simulink subsystem "ACC_Controller"  (R2024b)
settings: Solver=VariableStepAuto  StartTime=0.0  StopTime=10.0  RelTol=1e-3
libraries: mpcadaslib x1
settings Model: Creator=Tong  LastModifiedBy=Tong

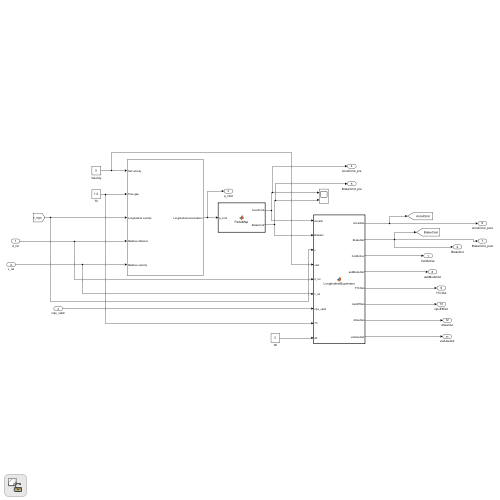
[thumbnail: Simulink's stored preview of the top-level diagram]
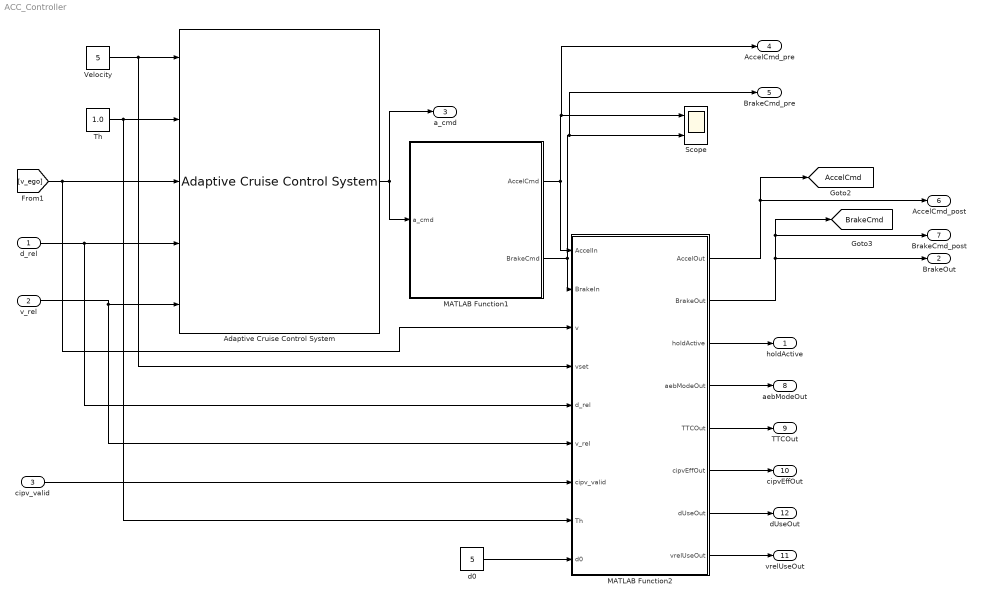
== system ACC_Controller ==
  d_rel : Inport
  v_rel : Inport  Port=2
  cipv_valid : Inport  Port=3
  Adaptive Cruise Control System : mpcadaslib/Adaptive Cruise Control System  EgoModel=tf(1,[0.5,1,0])  InitialEgoVelocity=5  DefaultSpacing=5  MaxVelocity=50  MinAcceleration=-2  amin_ext=off  MaxAcceleration=2  amax_ext=off  Ts=0.05  PredictionHorizon=30  ControllerBehavior=0.600  suboptimal=off  maxiter=10  datatypeopt=double  optmode=off  trackmode=off
      settings: LibrarySourceBlock=mpclib/Automated Driving/Adaptive Cruise Control System
  MATLAB Function1 : MATLAB Function  TreatAsAtomicUnit=on
  MATLAB Function2 : MATLAB Function  TreatAsAtomicUnit=on
  Scope : Scope  NumInputPorts=2
  Th : Constant  Value=1.0
  Velocity : Constant  Value=5
  d0 : Constant  Value=5
  holdActive : Outport
  BrakeOut : Outport  Port=2
  a_cmd : Outport  Port=3
  AccelCmd_pre : Outport  Port=4
  BrakeCmd_pre : Outport  Port=5
  AccelCmd_post : Outport  Port=6
  BrakeCmd_post : Outport  Port=7
  aebModeOut : Outport  Port=8
  TTCOut : Outport  Port=9
  cipvEffOut : Outport  Port=10
  vrelUseOut : Outport  Port=11
  dUseOut : Outport  Port=12
  tag scope: AccelCmd=global, BrakeCmd=global
  wires:
  d_rel/1 -> Adaptive Cruise Control System/4, MATLAB Function2/5(d_rel)
  v_rel/1 -> Adaptive Cruise Control System/5, MATLAB Function2/6(v_rel)
  [v_ego] -> Adaptive Cruise Control System/3, MATLAB Function2/3(v)
  Adaptive Cruise Control System/1 -> MATLAB Function1/1(a_cmd), a_cmd/1
  Th/1 -> Adaptive Cruise Control System/2, MATLAB Function2/8(Th)
  MATLAB Function1/1(AccelCmd) -> MATLAB Function2/1(AccelIn), Scope/1, AccelCmd_pre/1
  MATLAB Function1/2(BrakeCmd) -> MATLAB Function2/2(BrakeIn), Scope/2, BrakeCmd_pre/1
  MATLAB Function2/1(AccelOut) -> AccelCmd_post/1, [AccelCmd]
  MATLAB Function2/2(BrakeOut) -> BrakeOut/1, BrakeCmd_post/1, [BrakeCmd]
  Velocity/1 -> Adaptive Cruise Control System/1, MATLAB Function2/4(vset)
  d0/1 -> MATLAB Function2/9(d0)
  cipv_valid/1 -> MATLAB Function2/7(cipv_valid)
  MATLAB Function2/3(holdActive) -> holdActive/1
  MATLAB Function2/4(aebModeOut) -> aebModeOut/1
  MATLAB Function2/5(TTCOut) -> TTCOut/1
  MATLAB Function2/6(cipvEffOut) -> cipvEffOut/1
  MATLAB Function2/7(dUseOut) -> dUseOut/1
  MATLAB Function2/8(vrelUseOut) -> vrelUseOut/1

== matlab function ACC_Controller/MATLAB Function1 ==
  settings: updateMethod=DISCRETE
  data: a_cmd input; AccelCmd output; BrakeCmd output
function [AccelCmd, BrakeCmd] = PedalMap(a_cmd)
%#codegen
% a_cmd: desired longitudinal acceleration (m/s^2)
% outputs: AccelCmd/BrakeCmd in [0,1]

% === 需要按你的模型改的参数 ===
Ts = 0.05;        % 采样时间：与你Supervisor一致就行
aAccelMax = 2.0;  % 认为“满油门”对应的加速度 (m/s^2)
aBrakeMax = 4.0;  % 认为“满刹车”对应的减速度幅值 (m/s^2)
aDead = 0.08;     % 加速度死区 (m/s^2)，抑制0附近抖动：0.05~0.15可调

% 软启动非线性：>1 更温和（小命令更小踏板）
gammaAcc = 1.4;
gammaBrk = 1.2;

% 踏板变化率限制（每秒最大变化量）
pedalRate = 3.5;  % 1/s，越大越“灵”，越小越平顺（1.5~4可调）
dPed = pedalRate * Ts;

persistent accPrev brkPrev
if isempty(accPrev)
    accPrev = 0;
    brkPrev = 0;
end

% --- 1) 死区 + 归一化 ---
acc = 0;
brk = 0;

if a_cmd > aDead
    x = (a_cmd - aDead) / max(aAccelMax - aDead, 1e-3);
    x = min(max(x, 0), 1);
    acc = x^gammaAcc;
elseif a_cmd < -aDead
    x = (-a_cmd - aDead) / max(aBrakeMax - aDead, 1e-3);
    x = min(max(x, 0), 1);
    brk = x^gammaBrk;
end

% --- 2) 变化率限制（避免踏板突跳） ---
acc = min(max(acc, accPrev - dPed), accPrev + dPed);
brk = min(max(brk, brkPrev - dPed), brkPrev + dPed);

% --- 3) 互斥（稳妥，避免同时给油/给刹） ---
if brk > 0
    acc = 0;
elseif acc > 0
    brk = 0;
end

% --- 4) 限幅并更新 ---
AccelCmd = min(max(acc, 0), 1);
BrakeCmd = min(max(brk, 0), 1);

accPrev = AccelCmd;
brkPrev = BrakeCmd;
end

== matlab function ACC_Controller/MATLAB Function2 ==
  data: AccelIn input; AccelOut output; BrakeIn input; v input; vset input; d_rel input; v_rel input; cipv_valid input; Th input; d0 input; BrakeOut output; holdActive output; aebModeOut output; TTCOut output; cipvEffOut output; dUseOut output; vrelUseOut output
function [AccelOut, BrakeOut, holdActive, aebModeOut, TTCOut, cipvEffOut, dUseOut, vrelUseOut] = ...
    LongitudinalSupervisor(AccelIn, BrakeIn, v, vset, d_rel, v_rel, cipv_valid, Th, d0)
%#codegen
% LongitudinalSupervisor - Paper Mode
%
% 输入:
%   AccelIn, BrakeIn - 上游加速/制动命令，0~1
%   v                - ego 纵向速度，m/s
%   vset             - 设定速度，m/s
%   d_rel            - 真值相对距离，m
%   v_rel            - 真值相对速度，lead - ego，接近时为负
%   cipv_valid       - 上游目标有效标志
%   Th               - 时距
%   d0               - 最小间距
%
% 输出:
%   AccelOut, BrakeOut - 最终踏板命令
%   holdActive         - 停车保持状态
%   aebModeOut         - 0 none, 1 FCW, 2 PB1, 3 FB
%   TTCOut             - TTC
%   cipvEffOut         - Supervisor 实际采用的目标有效性
%   dUseOut            - Supervisor 实际使用距离
%   vrelUseOut         - Supervisor 实际使用相对速度

%% ================= 参数区 =================
TTC_MAX = 1e6;
NO_TARGET_DIST = 199.5;

% 论文模式：直接用真值距离/速度判断目标
USE_TRUTH_CONTROL = true;

% 目标丢失短时保持
Ts = 0.05;
t_drop_hold = 0.5;
N_drop = int32(round(t_drop_hold / Ts));

% ACC 安全距离
margin = 2.0;

% TTC 阈值
FCWtime = 1.8;
PB1time = 1.1;
FBtime  = 0.7;
TimeFactor = 1.3;
N_on = int32(2);

% 制动强度
PB1_brake = 0.25;
FB_brake  = 0.80;
EMG_brake = 1.00;

% 极近距离保护
d_emg = 1.5;

% 低速停车保持
v_hold = 0.25;
d_hold = d0 + 0.8;
d_relax = d0 + 2.0;
vrel_release = 0.15;

% 低速非紧急制动限幅，避免低速抖动太难看
v_low_brk_cap = 1.0;
brake_lowspd_cap = 0.45;

% 相对速度死区
if abs(v_rel) < 0.15
    v_rel = 0.0;
end

%% ================= 持久变量 =================
persistent haveLast lostCnt dLast vrelLast
persistent hold
persistent cntClosing aebMode

if isempty(haveLast)
    haveLast = false;
    lostCnt = int32(0);
    dLast = 200.0;
    vrelLast = 0.0;
end

if isempty(hold)
    hold = false;
end

if isempty(cntClosing)
    cntClosing = int32(0);
end

if isempty(aebMode)
    aebMode = int32(0);
end

%% ================= 1. 目标有效性与使用值 =================
if USE_TRUTH_CONTROL
    rawValid = (d_rel > 0.0) && (d_rel < NO_TARGET_DIST);

    if rawValid
        cipv_eff = true;
        d_use = d_rel;
        vrel_use = v_rel;

        haveLast = true;
        lostCnt = int32(0);
        dLast = d_use;
        vrelLast = vrel_use;
    else
        % 真值短时丢失时，保持上一帧，避免曲线突然跳 200
        if haveLast && (lostCnt < N_drop)
            lostCnt = lostCnt + 1;
            cipv_eff = true;
            d_use = dLast;
            vrel_use = vrelLast;
        else
            cipv_eff = false;
            d_use = 200.0;
            vrel_use = 0.0;

            haveLast = false;
            lostCnt = int32(0);
            dLast = 200.0;
            vrelLast = 0.0;
        end
    end
else
    % 原始模式：依赖 cipv_valid
    if cipv_valid > 0.5
        cipv_eff = true;
        d_use = d_rel;
        vrel_use = v_rel;

        haveLast = true;
        lostCnt = int32(0);
        dLast = d_use;
        vrelLast = vrel_use;
    else
        if haveLast && (lostCnt < N_drop)
            lostCnt = lostCnt + 1;
            cipv_eff = true;
            d_use = dLast;
            vrel_use = vrelLast;
        else
            cipv_eff = false;
            d_use = 200.0;
            vrel_use = 0.0;

            haveLast = false;
            lostCnt = int32(0);
        end
    end
end

%% ================= 2. 期望距离与 TTC =================
d_ref = d0 + Th * v;

closing = cipv_eff && (d_use > 0.0) && (vrel_use < -0.2) && (v > 0.3);

if closing
    TTC = d_use / (-vrel_use);
    if TTC > TTC_MAX
        TTC = TTC_MAX;
    end
else
    TTC = TTC_MAX;
end

TTCOut = TTC;

%% ================= 3. Stop & Hold =================
if (~hold) && cipv_eff && (v < v_hold) && (d_use < d_hold)
    hold = true;
end

if hold
    if (~cipv_eff) || ...
       ((vrel_use > vrel_release) && (d_use > d_relax)) || ...
       (d_use > d_ref + 1.0)
        hold = false;
    end
end

holdActive = hold;

%% ================= 4. AEB 状态机 =================
if closing && (TTC < FCWtime)
    cntClosing = min(cntClosing + 1, int32(100));
else
    cntClosing = int32(0);
end

closingStable = cntClosing >= N_on;

switch aebMode
    case 0
        if closingStable && (TTC < FCWtime)
            aebMode = int32(1);
        end

    case 1
        if (~closing) || (TTC > TimeFactor * FCWtime)
            aebMode = int32(0);
        elseif TTC < PB1time
            aebMode = int32(2);
        end

    case 2
        if (~closing) || (TTC > TimeFactor * PB1time)
            aebMode = int32(0);
        elseif TTC < FBtime
            aebMode = int32(3);
        end

    otherwise
        if (~closing) || (TTC > TimeFactor * FBtime)
            aebMode = int32(0);
        end
end

%% ================= 5. 输出优先级 =================
AccelOut = AccelIn;
BrakeOut = BrakeIn;

isEmergency = cipv_eff && (d_use < d_emg);

if isEmergency
    AccelOut = 0.0;
    BrakeOut = EMG_brake;

elseif hold
    AccelOut = 0.0;
    BrakeOut = EMG_brake;

else
    % AEB 分级
    if aebMode == 1
        AccelOut = 0.0;

    elseif aebMode == 2
        AccelOut = 0.0;
        if BrakeOut < PB1_brake
            BrakeOut = PB1_brake;
        end

    elseif aebMode == 3
        AccelOut = 0.0;
        if BrakeOut < FB_brake
            BrakeOut = FB_brake;
        end
    end

    % 安全距离内且正在接近：禁止继续加速
    if cipv_eff && (d_use < d_ref + margin) && (vrel_use < -0.1)
        AccelOut = 0.0;

        % 给一点温和制动，让图上能体现监督层介入
        if BrakeOut < 0.10
            BrakeOut = 0.10;
        end
    end

    % 没有目标时，不主动覆盖上游制动；只防止小残余刹车长期存在
    if (~cipv_eff) && (BrakeOut < 0.03)
        BrakeOut = 0.0;
    end

    % 低速下非 FB 不要太猛
    if (v < v_low_brk_cap) && (aebMode < 3) && (~isEmergency)
        if BrakeOut > brake_lowspd_cap
            BrakeOut = brake_lowspd_cap;
        end
    end
end

%% ================= 6. 加速制动互斥 =================
if (BrakeOut > 0.001) && (AccelOut > 0.001)
    if BrakeOut >= AccelOut
        AccelOut = 0.0;
    else
        BrakeOut = 0.0;
    end
end

%% ================= 7. 限幅 =================
if AccelOut < 0.0
    AccelOut = 0.0;
elseif AccelOut > 1.0
    AccelOut = 1.0;
end

if BrakeOut < 0.0
    BrakeOut = 0.0;
elseif BrakeOut > 1.0
    BrakeOut = 1.0;
end

%% ================= 8. 日志输出 =================
aebModeOut = double(aebMode);
cipvEffOut = double(cipv_eff);
dUseOut = d_use;
vrelUseOut = vrel_use;

end


% function [AccelOut, BrakeOut, holdActive, aebModeOut, TTCOut, cipvEffOut, dUseOut, vrelUseOut] = ...
%     LongitudinalSupervisor(AccelIn, BrakeIn, v, vset, d_rel, v_rel, cipv_valid, Th, d0)
% %#codegen
% % LongitudinalSupervisor (0~1 pedal commands)
% % v_rel 定义：lead - ego（接近时 v_rel<0）
% 
% %% ========== 采样时间 ==========
% Ts = 0.05;
% 
% %% ========== 参数区（可调） ==========
% epsV   = 0.2;
% margin = 2.0;
% K_over = 0.35;
% 
% v_hold       = 0.3;
% d_hold       = d0 + 0.8;
% d_relax      = d0 + 2.0;
% vrel_release = 0.15;
% relax_by_ref = 1.0;
% 
% d_emg = 1.5;
% 
% t_drop_hold = 0.5;
% N_drop = int32(round(t_drop_hold/Ts));
% 
% v_low_brk_cap    = 1.0;
% brake_lowspd_cap = 0.35;
% 
% if abs(v_rel) < 0.2
%     v_rel = 0;
% end
% 
% FCWtime    = 1.8;
% PB1time    = 1.1;
% FBtime     = 0.7;
% TimeFactor = 1.3;
% N_on       = int32(3);
% PB1_brake_min = 0.15;
% 
% %% ========== 期望距离 ==========
% d_ref = d0 + Th*v;
% 
% %% ========== 目标丢失保持 ==========
% persistent lostCnt haveLast dLast vrelLast
% if isempty(haveLast)
%     lostCnt  = int32(0);
%     haveLast = false;
%     dLast    = 200;
%     vrelLast = 0;
% end
% 
% if cipv_valid > 0.5
%     haveLast = true;
%     lostCnt  = int32(0);
%     dLast    = d_rel;
%     vrelLast = v_rel;
%     cipv_eff = true;
%     d_use    = d_rel;
%     vrel_use = v_rel;
% else
%     if haveLast && (lostCnt < N_drop)
%         lostCnt  = lostCnt + 1;
%         cipv_eff = true;
%         d_use    = dLast;
%         vrel_use = vrelLast;
%     else
%         cipv_eff = false;
%         d_use    = d_rel;
%         vrel_use = v_rel;
%         haveLast = false;
%     end
% end
% 
% %% ========== Stop&Hold 状态机 ==========
% persistent hold
% if isempty(hold), hold = false; end
% 
% if (~hold) && cipv_eff && (v < v_hold) && (d_use < d_hold)
%     hold = true;
% end
% 
% if hold
%     if (~cipv_eff) || ...
%        ((vrel_use > vrel_release) && (d_use > d_relax)) || ...
%        (d_use > d_ref + relax_by_ref)
%         hold = false;
%     end
% end
% 
% holdActive = hold;
% 
% %% ========== TTC分级状态机 ==========
% closing = cipv_eff && (vrel_use < -0.2) && (d_use > 0) && (v > 0.5);
% % if closing
% %     TTC = d_use / (-vrel_use);
% % else
% %     TTC = inf;
% % end
% 
% TTC_MAX = 1e6;
% if closing && (-vrel_use > 1e-3)
%     TTC = d_use / (-vrel_use);
%     if TTC > TTC_MAX
%         TTC = TTC_MAX;
%     end
% else
%     TTC = TTC_MAX;
% end
% TTCOut = TTC;
% 
% persistent cntClosing aebMode
% if isempty(cntClosing), cntClosing = int32(0); end
% if isempty(aebMode),    aebMode    = int32(0); end
% % aebMode: 0 Default, 1 FCW, 2 PB1, 3 FB
% 
% if closing && (TTC < FCWtime)
%     cntClosing = min(cntClosing + 1, int32(100));
% else
%     cntClosing = int32(0);
% end
% closingStable = (cntClosing >= N_on);
% 
% switch aebMode
%     case 0
%         if closingStable && (TTC < FCWtime)
%             aebMode = int32(1);
%         end
%     case 1
%         if (~closing) || (TTC > TimeFactor*FCWtime)
%             aebMode = int32(0);
%         elseif TTC < PB1time
%             aebMode = int32(2);
%         end
%     case 2
%         if (~closing) || (TTC > TimeFactor*PB1time)
%             aebMode = int32(0);
%         elseif TTC < FBtime
%             aebMode = int32(3);
%         end
%     otherwise % 3
%         if (~closing) || (TTC > TimeFactor*FBtime)
%             aebMode = int32(0);
%         end
% end
% 
% %% ========== 默认继承上游 ==========
% AccelOut = AccelIn;
% BrakeOut = BrakeIn;
% 
% %% ========== 优先级逻辑 ==========
% isEmergency = cipv_eff && (d_use < d_emg);
% 
% if isEmergency
%     AccelOut = 0;
%     BrakeOut = 1.0;
% 
% elseif hold
%     AccelOut = 0;
%     BrakeOut = 1.0;
% 
% else
%     if aebMode == 1
%         AccelOut = 0;
%     elseif aebMode == 2
%         AccelOut = 0;
%         BrakeOut = max(BrakeOut, PB1_brake_min);
%     elseif aebMode == 3
%         AccelOut = 0;
%         BrakeOut = 1.0;
%     end
% 
%     % if v > vset + epsV
%     %     AccelOut = 0;
%     %     BrakeOut = max(BrakeOut, min(1.0, K_over*(v - vset)));
%     % end
% 
%     if cipv_eff && (d_use < d_ref + margin) && (vrel_use < -0.1)
%         AccelOut = 0;
%     end
% 
%     if (~cipv_eff) && (v <= vset + epsV)
%         BrakeOut = 0;
%     end
% 
%     if (v < v_low_brk_cap) && (aebMode < 3)
%         BrakeOut = min(BrakeOut, brake_lowspd_cap);
%     end
% end
% 
% %% ========== 互斥 ==========
% if (BrakeOut > 0) && (AccelOut > 0)
%     if BrakeOut >= AccelOut
%         AccelOut = 0;
%     else
%         BrakeOut = 0;
%     end
% end
% 
% %% ========== 限幅 ==========
% AccelOut = min(max(AccelOut, 0), 1);
% BrakeOut = min(max(BrakeOut, 0), 1);
% 
% %% ========== 新增日志输出 ==========
% aebModeOut = double(aebMode);   % 便于To Workspace/Scope记录
% TTCOut     = TTC;
% cipvEffOut = double(cipv_eff);
% dUseOut    = d_use;
% vrelUseOut = vrel_use;
% 
% end


% function [AccelOut, BrakeOut, holdActive] = LongitudinalSupervisor(AccelIn, BrakeIn, v, vset, d_rel, v_rel, cipv_valid, Th, d0)
% %#codegen
% % LongitudinalSupervisor (0~1 pedal commands)
% % v_rel 定义：lead - ego（接近时 v_rel<0）
% 
% %% ========== 采样时间 ==========
% Ts = 0.05;   % 如果你的Supervisor不是0.05s，改这里
% 
% %% ========== 参数区（可调） ==========
% % 通用
% epsV   = 0.2;     % 超速带 (m/s)
% margin = 2.0;     % 接近期望距离的裕度 (m)
% K_over = 0.35;     % 超速刹车增益（0~1映射前的强度）
% 
% % Stop&Hold
% v_hold      = 0.3;         % 认为停住
% d_hold      = d0 + 0.8;    % 进入hold（跟d0绑定）
% d_relax     = d0 + 2.0;    % 退出hold滞回
% vrel_release = 0.3;        % 前车确实在拉开（v_rel>0）
% 
% % 极限兜底（非常近距离强制全刹）
% d_emg = 1.5;   % gap小于此值 -> 全刹（最后保险）
% 
% % 丢目标保持（防cipv_valid抖动）
% t_drop_hold = 0.5;                 % s
% N_drop = int32(round(t_drop_hold/Ts));
% 
% % v_rel死区（抑制差分噪声）
% if abs(v_rel) < 0.2
%     v_rel = 0;
% end
% 
% % === TTC 分级（模仿demo）===
% % 阈值含义：TTC 小于阈值 -> 更危险
% FCWtime = 1.8;   % 进入FCW：禁止继续给油（不强制刹）
% PB1time = 1.1;   % 进入PB1：部分制动
% FBtime  = 0.7;   % 进入FB ：全制动（强制刹）
% TimeFactor = 1.3; % 退出滞回：阈值*TimeFactor 才退出，防抖
% 
% % 进入稳定帧数（Ts=0.05时，3帧=0.15s）
% N_on = int32(3);
% 
% % 制动档位对应的最小刹车开度（0~1）
% PB1_brake_min = 0.15;  % 部分制动（你觉得刹得太猛就调小到0.15~0.2）
% % FB 直接 1.0
% 
% %% ========== 期望距离 ==========
% d_ref = d0 + Th*v;
% 
% %% ========== 目标丢失保持：生成 cipv_eff + d_use/vrel_use ==========
% persistent lostCnt haveLast dLast vrelLast
% if isempty(haveLast)
%     lostCnt  = int32(0);
%     haveLast = false;
%     dLast    = 200;
%     vrelLast = 0;
% end
% 
% if cipv_valid > 0.5
%     haveLast = true;
%     lostCnt  = int32(0);
%     dLast    = d_rel;
%     vrelLast = v_rel;
%     cipv_eff = true;
%     d_use    = d_rel;
%     vrel_use = v_rel;
% else
%     if haveLast && (lostCnt < N_drop)
%         lostCnt  = lostCnt + 1;
%         cipv_eff = true;
%         d_use    = dLast;
%         vrel_use = vrelLast;
%     else
%         cipv_eff = false;
%         d_use    = d_rel;
%         vrel_use = v_rel;
%         haveLast = false;
%     end
% end
% 
% %% ========== Stop&Hold 状态机 ==========
% persistent hold
% if isempty(hold), hold = false; end
% 
% % 进入 hold：有目标、停住、距离够近
% % if (~hold) && cipv_eff && (v < v_hold) && (d_use < d_hold)
% %     hold = true;
% % end
% if (~hold) && cipv_eff && (v < v_hold) && (d_use < d_hold)
%     hold = true;
% end
% 
% % 退出 hold：目标真丢失 或 前车确实走了且距离超过滞回
% if hold
%     if (~cipv_eff) || ((vrel_use > vrel_release) && (d_use > d_relax))
%         hold = false;
%     end
% end
% 
% holdActive = hold;
% 
% %% ========== TTC + 分级制动状态机（模仿demo） ==========
% % TTC 定义：只在接近时有效（vrel_use<0）
% closing = cipv_eff && (vrel_use < -0.2) && (d_use > 0) && (v > 0.5);
% if closing
%     TTC = d_use / (-vrel_use);  % 秒，越小越危险
% else
%     TTC = inf;
% end
% 
% % 连续帧稳定判定（避免一次噪声触发）
% persistent cntClosing aebMode
% if isempty(cntClosing), cntClosing = int32(0); end
% if isempty(aebMode),    aebMode = int32(0);    end
% % aebMode: 0 Default, 1 FCW, 2 PB1, 3 FB
% 
% if closing && (TTC < FCWtime)
%     cntClosing = min(cntClosing + 1, int32(100));
% else
%     cntClosing = int32(0);
% end
% closingStable = (cntClosing >= N_on);
% 
% switch aebMode
%     case 0 % Default
%         if closingStable && (TTC < FCWtime)
%             aebMode = int32(1);
%         end
% 
%     case 1 % FCW
%         if (~closing) || (TTC > TimeFactor*FCWtime)
%             aebMode = int32(0);
%         elseif TTC < PB1time
%             aebMode = int32(2);
%         end
% 
%     case 2 % PB1
%         if (~closing) || (TTC > TimeFactor*PB1time)
%             aebMode = int32(0);
%         elseif TTC < FBtime
%             aebMode = int32(3);
%         end
% 
%     otherwise % 3 FB
%         if (~closing) || (TTC > TimeFactor*FBtime)
%             aebMode = int32(0);
%         end
% end
% 
% %% ========== 默认继承上游 ==========
% AccelOut = AccelIn;
% BrakeOut = BrakeIn;
% 
% %% ========== 最高优先级：极限距离兜底 ==========
% if cipv_eff && (d_use < d_emg)
%     AccelOut = 0;
%     BrakeOut = 1.0;
% 
% %% ========== Stop&Hold（抱死防蠕动） ==========
% elseif hold
%     AccelOut = 0;
%     BrakeOut = 1.0;
% 
% else
%     %% ========== TTC分级覆盖层（模仿demo） ==========
%     % 注意：它是“覆盖/钳制”，只会更保守
%     if aebMode == 1
%         % FCW：禁止继续给油
%         AccelOut = 0;
% 
%     elseif aebMode == 2
%         % PB1：部分制动
%         AccelOut = 0;
%         BrakeOut = max(BrakeOut, PB1_brake_min);
% 
%     elseif aebMode == 3
%         % FB：全制动
%         AccelOut = 0;
%         BrakeOut = 1.0;
%     end
% 
%     %% ========== 超速抑制（下坡也压住） ==========
%     % if v > vset + epsV
%     %     AccelOut = 0;
%     %     BrakeOut = max(BrakeOut, min(1.0, K_over*(v - vset)));
%     % end
% 
%     %% ========== 接近期望距离：禁止继续给油（防蠕动/顶着前车） ==========
%     % if cipv_eff && (d_use < d_ref + margin)
%     %     AccelOut = 0;
%     % end
%     if cipv_eff && (d_use < d_ref + margin) && (vrel_use < -0.1)
%         AccelOut = 0;
%     end
% 
%     %% ========== 无目标且未超速：禁止“鬼刹车” ==========
%     % if (~cipv_eff) && (v <= vset + epsV)
%     %     BrakeOut = 0;
%     % end
% end
% 
% %% ========== 油门/刹车互斥（谁大留谁） ==========
% if (BrakeOut > 0) && (AccelOut > 0)
%     if BrakeOut >= AccelOut
%         AccelOut = 0;
%     else
%         BrakeOut = 0;
%     end
% end
% 
% %% ========== 限幅 ==========
% AccelOut = min(max(AccelOut, 0), 1);
% BrakeOut = min(max(BrakeOut, 0), 1);
% 
% end


% function [AccelOut, BrakeOut, holdActive] = LongitudinalSupervisor(AccelIn, BrakeIn, v, vset, d_rel, v_rel, cipv_valid, Th, d0)
% %#codegen
% 
% % === 如果你的采样时间不是0.05，改这里 ===
% Ts = 0.01;
% 
% % ===== 参数 =====
% epsV   = 0.2;
% margin = 2.0;
% 
% d_emg = 1.5;     % 紧急刹车阈值(gap)
% 
% v_hold = 0.3;    % 认为停住
% % 关键：hold阈值跟 d0 绑定（避免停在d0附近不hold导致蠕动）
% d_hold  = d0 + 0.8;   % 建议 d0+0.5 ~ d0+1.5
% d_relax = d0 + 2.0;   % 滞回：比进入大 1~2m
% 
% % 退出hold需要前车“确实走了”
% vrel_release = 0.3;   % v_rel=lead-ego (你TruthRel是 leadV-egoV)，>0 表示前车在拉开
% K_over  = 0.6;
% 
% % 丢目标保持时间：避免cipv_valid抖动导致松刹
% t_drop_hold = 0.5;                 % s
% N_drop = int32(round(t_drop_hold/Ts));
% % =================
% 
% % v_rel 死区（抑制差分噪声导致的误动作）
% if abs(v_rel) < 0.2
%     v_rel = 0;
% end
% 
% d_ref = d0 + Th*v;
% 
% % ---------- 目标丢失保持：生成 cipv_eff + d_use/vrel_use ----------
% persistent lostCnt haveLast dLast vrelLast
% if isempty(haveLast)
%     lostCnt = int32(0);
%     haveLast = false;
%     dLast = 200;
%     vrelLast = 0;
% end
% 
% if cipv_valid
%     haveLast = true;
%     lostCnt = int32(0);
%     dLast = d_rel;
%     vrelLast = v_rel;
%     cipv_eff = true;
%     d_use = d_rel;
%     vrel_use = v_rel;
% else
%     if haveLast && (lostCnt < N_drop)
%         lostCnt = lostCnt + 1;
%         cipv_eff = true;      % 短时仍当“有目标”
%         d_use = dLast;        % 用上一次有效值做逻辑
%         vrel_use = vrelLast;
%     else
%         cipv_eff = false;
%         d_use = d_rel;
%         vrel_use = v_rel;
%         haveLast = false;
%     end
% end
% % ----------------------------------------------------------------
% 
% % ---------- Stop&Hold 状态机（用 cipv_eff 和 d_use） ----------
% persistent hold
% if isempty(hold), hold = false; end
% 
% % 进入 hold：有目标、停住、距离进入阈值
% if (~hold) && cipv_eff && (v < v_hold) && (d_use < d_hold)
%     hold = true;
% end
% 
% % 退出 hold：目标真丢失 / 前车开始拉开且距离超过滞回
% if hold
%     if (~cipv_eff) || ((vrel_use > vrel_release) && (d_use > d_relax))
%         hold = false;
%     end
% end
% holdActive = hold;
% % ----------------------------------------------------------------
% 
% % 默认继承上游
% AccelOut = AccelIn;
% BrakeOut = BrakeIn;
% 
% % 1) 紧急制动（优先级最高）
% if cipv_eff && (d_use < d_emg)
%     AccelOut = 0;
%     BrakeOut = 1;
% 
% % 2) Stop&Hold：停住抱死，消除蠕动
% elseif hold
%     AccelOut = 0;
%     BrakeOut = 1;
% 
% else
%     % 3) 超速抑制：下坡也压住
%     if v > vset + epsV
%         AccelOut = 0;
%         BrakeOut = max(BrakeOut, min(1, K_over*(v - vset)));
%     end
% 
%     % 4) 接近期望距离：禁止继续给油（防蠕动）
%     if cipv_eff && (d_use < d_ref + margin)
%         AccelOut = 0;
%     end
% 
%     % 5) 无目标且未超速：禁止鬼刹车
%     if (~cipv_eff) && (v <= vset + epsV)
%         BrakeOut = 0;
%     end
% end
% 
% % 6) 纵向互斥（更温和的互斥：谁大留谁）
% if (BrakeOut > 0) && (AccelOut > 0)
%     if BrakeOut >= AccelOut
%         AccelOut = 0;
%     else
%         BrakeOut = 0;
%     end
% end
% 
% % 限幅
% AccelOut = min(max(AccelOut,0),1);
% BrakeOut = min(max(BrakeOut,0),1);
% end

% function [AccelOut, BrakeOut] = BrakeGuard(AccelIn, BrakeIn, v, vset, d_rel, cipv_valid, Th, d0)
% %#codegen
% epsV = 0.2;     % 超速带
% margin = 2.0;   % 距离裕度
% 
% d_ref = d0 + Th*v;
% 
% allowBrake = false;
% 
% % 超速允许刹（下坡也能压住）
% if v > vset + epsV
%     allowBrake = true;
% end
% 
% % 有前车且距离过近允许刹
% if cipv_valid && (d_rel < d_ref + margin)
%     allowBrake = true;
% end
% 
% AccelOut = AccelIn;
% if allowBrake
%     BrakeOut = BrakeIn;
% else
%     BrakeOut = 0;
% end
% end



% function [AccelOut, BrakeOut] = LongitudinalSupervisor(AccelIn, BrakeIn, v, vset, d_rel, v_rel, cipv_valid, Th, d0)
% %#codegen
% % LongitudinalSupervisor
% % 纵向监督层（合并版）：
% % 1) 禁止鬼刹车（无前车且未超速时不允许刹车）
% % 2) 超速抑制（下坡也能压住速度）
% % 3) 紧急制动（距离过小强制全刹）
% % 4) Stop&Hold（低速近距离保持刹车，消除蠕动）
% % 5) 反蠕动（距离接近 d_ref 时禁止继续给油）
% 
% % ---------------- 参数区（先用默认，后面再调） ----------------
% epsV   = 0.2;    % 超速带 (m/s)
% margin = 2.0;    % 跟车距离裕度 (m)
% 
% d_emg   = 1.5;   % 紧急刹车阈值（gap，小于这个全刹）
% d_hold  = 2.5;   % 进入停车保持的距离阈值
% d_relax = 3.5;   % 退出停车保持的距离阈值（滞回）
% v_hold  = 0.3;   % 判定停住的速度阈值 (m/s)
% 
% K_over  = 0.5;   % 超速刹车增益（越大刹得越猛）
% % --------------------------------------------------------------
% 
% % 期望距离
% d_ref = d0 + Th*v;
% 
% % 估计前车沿前向速度（假设 v_rel = v_lead_long - v）
% v_lead_long = v_rel + v;
% 
% % 默认继承上游命令
% AccelOut = AccelIn;
% BrakeOut = BrakeIn;
% 
% % ---------------- Stop&Hold 状态机 ----------------
% persistent hold
% if isempty(hold)
%     hold = false;
% end
% 
% % 进入 hold：有前车、距离近、且基本停住
% if (~hold) && cipv_valid && (d_rel < d_hold) && (v < v_hold)
%     hold = true;
% end
% 
% % 退出 hold：目标无效 / 距离拉开 / 前车开始走
% if hold
%     if (~cipv_valid) || (d_rel > d_relax) || (v_lead_long > 0.5)
%         hold = false;
%     end
% end
% % ---------------------------------------------------
% 
% % 1) 紧急制动：gap 太小，直接全刹（最高优先级）
% if cipv_valid && (d_rel < d_emg)
%     AccelOut = 0;
%     BrakeOut = 1;
%     return;
% end
% 
% % 2) Stop&Hold：保持刹车，消除刹停后蠕动
% if hold
%     AccelOut = 0;
%     BrakeOut = 1;
%     return;
% end
% 
% % 3) 超速抑制：超速时禁止给油，并且允许/增加刹车
% if v > vset + epsV
%     AccelOut = 0;
%     BrakeOut = max(BrakeOut, min(1, K_over*(v - vset)));
%     return;
% end
% 
% % 4) 跟车反蠕动：接近期望距离时禁止继续给油（让上游决定是否轻刹）
% if cipv_valid && (d_rel < d_ref + margin)
%     AccelOut = 0;
% end
% 
% % 5) 禁止鬼刹车：无前车且不超速时不允许刹车
% if (~cipv_valid) && (v <= vset + epsV)
%     BrakeOut = 0;
% end
% 
% % 6) 输出限幅（稳妥）
% if AccelOut < 0, AccelOut = 0; end
% if AccelOut > 1, AccelOut = 1; end
% if BrakeOut < 0, BrakeOut = 0; end
% if BrakeOut > 1, BrakeOut = 1; end
% end



% function [AccelOut, BrakeOut, holdActive] = LongitudinalSupervisor(AccelIn, BrakeIn, v, vset, d_rel, v_rel, cipv_valid, Th, d0)
% %#codegen
% 
% % ===== 参数 =====
% epsV   = 0.2;
% margin = 2.0;
% 
% d_emg   = 1.5;   % 紧急刹车阈值(gap)
% d_hold  = 2.5;   % 进入hold
% d_relax = 3.5;   % 退出hold
% v_hold  = 0.3;   % 认为停住
% 
% K_over  = 0.6;   % 超速刹车增益
% % ===============
% 
% d_ref = d0 + Th*v;
% 
% % 前车纵向速度估计（假设 v_rel = v_lead_long - v）
% v_lead_long = v_rel + v;
% 
% persistent hold
% if isempty(hold), hold = false; end
% 
% % --- 进入/退出 hold（只在有前车时生效）---
% if (~hold) && cipv_valid && (d_rel < d_hold) && (v < v_hold)
%     hold = true;
% end
% if hold
%     if (~cipv_valid) || (d_rel > d_relax) || (v_lead_long > 0.5)
%         hold = false;
%     end
% end
% holdActive = hold;
% 
% % 默认继承上游
% AccelOut = AccelIn;
% BrakeOut = BrakeIn;
% 
% % 1) 紧急制动（gap过小）
% if cipv_valid && (d_rel < d_emg)
%     AccelOut = 0;
%     BrakeOut = 1;
% else
%     % 2) Stop&Hold：有前车且停住 -> 抱死
%     if hold
%         AccelOut = 0;
%         BrakeOut = 1;
%     else
%         % 3) 超速抑制：下坡也压住
%         if v > vset + epsV
%             AccelOut = 0;
%             BrakeOut = max(BrakeOut, min(1, K_over*(v - vset)));
%         end
% 
%         % 4) 跟车接近时禁止继续给油（防蠕动）
%         if cipv_valid && (d_rel < d_ref + margin)
%             AccelOut = 0;
%         end
% 
%         % 5) 无前车且未超速：禁止鬼刹车
%         if (~cipv_valid) && (v <= vset + epsV)
%             BrakeOut = 0;
%         end
%     end
% end
% 
% % 6) 纵向互斥（关键：绝不允许同时给油和给刹）
% if BrakeOut > 0
%     AccelOut = 0;
% end
% if AccelOut > 0
%     BrakeOut = 0;
% end
% 
% % 限幅
% AccelOut = min(max(AccelOut,0),1);
% BrakeOut = min(max(BrakeOut,0),1);
% end
